simulink subsystem "offset_triangle_wave"  (R2023b)
settings: Solver=VariableStepAuto  StartTime=0.0  StopTime=10.0  RelTol=1e-3
model mask{offset=0, gain=0, freq=100}
libraries: spsTriangleGeneratorLib x1
settings Model: Creator=javeed  LastModifiedBy=USER
settings RTWCC: GPUComputeCapability=5.0

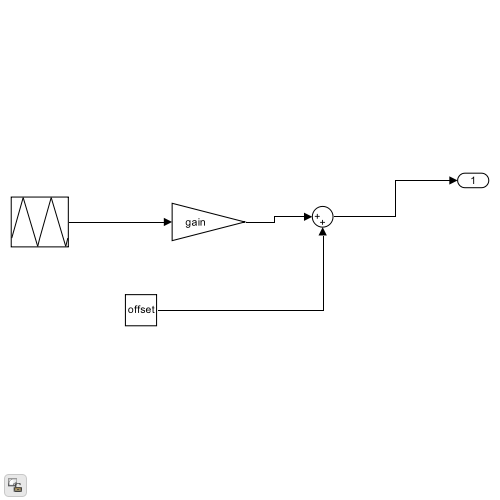
[thumbnail: Simulink's stored preview of the top-level diagram]
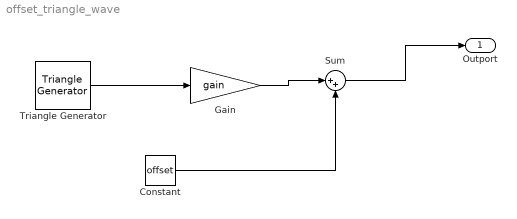
== system offset_triangle_wave ==
  Constant : Constant  Value=offset
  Gain : Gain  Gain=gain
  Sum : Sum  Inputs=|++
  Triangle Generator : spsTriangleGeneratorLib/Triangle Generator  Freq=50  Phase=30  Ts=0
  Outport : Outport
  wires:
  Constant/1 -> Sum/2
  Triangle Generator/1 -> Gain/1
  Gain/1 -> Sum/1
  Sum/1 -> Outport/1
